simulink model "PeakDetect3"  (R2018b)
settings: Solver=FixedStepAuto  StartTime=0  StopTime=500*(15e-9)  FixedStep=15e-9  RelTol=1e-3
libraries: simulink x35, hdlsllib x34
(part 4 of 4)

== system PeakDetect3/xcorr_q1/Subsystem/Enabled Subsystem124 ==
  In1 : Inport
  Enable : EnablePort
  Out1 : Outport  InitialOutput=0
  wires:
  In1/1 -> Out1/1

== system PeakDetect3/xcorr_q1/Subsystem/Enabled Subsystem125 ==
  In1 : Inport
  Enable : EnablePort
  Out1 : Outport  InitialOutput=0
  wires:
  In1/1 -> Out1/1

== system PeakDetect3/xcorr_q1/Subsystem/Enabled Subsystem126 ==
  In1 : Inport
  Enable : EnablePort
  Out1 : Outport  InitialOutput=0
  wires:
  In1/1 -> Out1/1

== system PeakDetect3/xcorr_q1/Subsystem/Enabled Subsystem127 ==
  In1 : Inport
  Enable : EnablePort
  Out1 : Outport  InitialOutput=0
  wires:
  In1/1 -> Out1/1

== system PeakDetect3/xcorr_q1/Subsystem/Enabled Subsystem128 ==
  In1 : Inport
  Enable : EnablePort
  Out1 : Outport  InitialOutput=0
  wires:
  In1/1 -> Out1/1

== system PeakDetect3/xcorr_q1/Subsystem/Enabled Subsystem129 ==
  In1 : Inport
  Enable : EnablePort
  Out1 : Outport  InitialOutput=0
  wires:
  In1/1 -> Out1/1

== system PeakDetect3/xcorr_q1/Subsystem/Enabled Subsystem130 ==
  In1 : Inport
  Enable : EnablePort
  Out1 : Outport  InitialOutput=0
  wires:
  In1/1 -> Out1/1

== system PeakDetect3/xcorr_q1/Subsystem/Enabled Subsystem131 ==
  In1 : Inport
  Enable : EnablePort
  Out1 : Outport  InitialOutput=0
  wires:
  In1/1 -> Out1/1

== system PeakDetect3/xcorr_q1/Subsystem/Enabled Subsystem132 ==
  In1 : Inport
  Enable : EnablePort
  Out1 : Outport  InitialOutput=0
  wires:
  In1/1 -> Out1/1

== system PeakDetect3/xcorr_q1/Subsystem/Enabled Subsystem133 ==
  In1 : Inport
  Enable : EnablePort
  Out1 : Outport  InitialOutput=0
  wires:
  In1/1 -> Out1/1

== system PeakDetect3/xcorr_q1/Subsystem/Enabled Subsystem134 ==
  In1 : Inport
  Enable : EnablePort
  Out1 : Outport  InitialOutput=0
  wires:
  In1/1 -> Out1/1

== system PeakDetect3/xcorr_q1/Subsystem/Enabled Subsystem135 ==
  In1 : Inport
  Enable : EnablePort
  Out1 : Outport  InitialOutput=0
  wires:
  In1/1 -> Out1/1

== system PeakDetect3/xcorr_q1/Subsystem/Enabled Subsystem136 ==
  In1 : Inport
  Enable : EnablePort
  Out1 : Outport  InitialOutput=0
  wires:
  In1/1 -> Out1/1

== system PeakDetect3/xcorr_q1/Subsystem/Enabled Subsystem137 ==
  In1 : Inport
  Enable : EnablePort
  Out1 : Outport  InitialOutput=0
  wires:
  In1/1 -> Out1/1

== system PeakDetect3/xcorr_q1/Subsystem/Enabled Subsystem138 ==
  In1 : Inport
  Enable : EnablePort
  Out1 : Outport  InitialOutput=0
  wires:
  In1/1 -> Out1/1

== system PeakDetect3/xcorr_q1/Subsystem/Enabled Subsystem139 ==
  In1 : Inport
  Enable : EnablePort
  Out1 : Outport  InitialOutput=0
  wires:
  In1/1 -> Out1/1

== system PeakDetect3/xcorr_q1/Subsystem/Enabled Subsystem140 ==
  In1 : Inport
  Enable : EnablePort
  Out1 : Outport  InitialOutput=0
  wires:
  In1/1 -> Out1/1

== system PeakDetect3/xcorr_q1/Subsystem/Enabled Subsystem141 ==
  In1 : Inport
  Enable : EnablePort
  Out1 : Outport  InitialOutput=0
  wires:
  In1/1 -> Out1/1

== system PeakDetect3/xcorr_q1/Subsystem/Enabled Subsystem142 ==
  In1 : Inport
  Enable : EnablePort
  Out1 : Outport  InitialOutput=0
  wires:
  In1/1 -> Out1/1

== system PeakDetect3/xcorr_q1/Subsystem/Enabled Subsystem143 ==
  In1 : Inport
  Enable : EnablePort
  Out1 : Outport  InitialOutput=0
  wires:
  In1/1 -> Out1/1

== system PeakDetect3/xcorr_q1/Subsystem/Enabled Subsystem144 ==
  In1 : Inport
  Enable : EnablePort
  Out1 : Outport  InitialOutput=0
  wires:
  In1/1 -> Out1/1

== system PeakDetect3/xcorr_q1/Subsystem/Enabled Subsystem145 ==
  In1 : Inport
  Enable : EnablePort
  Out1 : Outport  InitialOutput=0
  wires:
  In1/1 -> Out1/1

== system PeakDetect3/xcorr_q1/Subsystem/Enabled Subsystem146 ==
  In1 : Inport
  Enable : EnablePort
  Out1 : Outport  InitialOutput=0
  wires:
  In1/1 -> Out1/1

== system PeakDetect3/xcorr_q1/Subsystem/Enabled Subsystem147 ==
  In1 : Inport
  Enable : EnablePort
  Out1 : Outport  InitialOutput=0
  wires:
  In1/1 -> Out1/1

== system PeakDetect3/xcorr_q1/Subsystem/Enabled Subsystem148 ==
  In1 : Inport
  Enable : EnablePort
  Out1 : Outport  InitialOutput=0
  wires:
  In1/1 -> Out1/1

== system PeakDetect3/xcorr_q1/Subsystem/Enabled Subsystem149 ==
  In1 : Inport
  Enable : EnablePort
  Out1 : Outport  InitialOutput=0
  wires:
  In1/1 -> Out1/1

== system PeakDetect3/xcorr_q1/Subsystem/Enabled Subsystem150 ==
  In1 : Inport
  Enable : EnablePort
  Out1 : Outport  InitialOutput=0
  wires:
  In1/1 -> Out1/1

== system PeakDetect3/xcorr_q1/Subsystem/Enabled Subsystem151 ==
  In1 : Inport
  Enable : EnablePort
  Out1 : Outport  InitialOutput=0
  wires:
  In1/1 -> Out1/1

== system PeakDetect3/xcorr_q1/Subsystem/Enabled Subsystem152 ==
  In1 : Inport
  Enable : EnablePort
  Out1 : Outport  InitialOutput=0
  wires:
  In1/1 -> Out1/1

== system PeakDetect3/xcorr_q1/Subsystem/Enabled Subsystem153 ==
  In1 : Inport
  Enable : EnablePort
  Out1 : Outport  InitialOutput=0
  wires:
  In1/1 -> Out1/1

== system PeakDetect3/xcorr_q1/Subsystem/Enabled Subsystem154 ==
  In1 : Inport
  Enable : EnablePort
  Out1 : Outport  InitialOutput=0
  wires:
  In1/1 -> Out1/1

== system PeakDetect3/xcorr_q1/Subsystem/Enabled Subsystem155 ==
  In1 : Inport
  Enable : EnablePort
  Out1 : Outport  InitialOutput=0
  wires:
  In1/1 -> Out1/1

== system PeakDetect3/xcorr_q1/Subsystem/Enabled Subsystem156 ==
  In1 : Inport
  Enable : EnablePort
  Out1 : Outport  InitialOutput=0
  wires:
  In1/1 -> Out1/1

== system PeakDetect3/xcorr_q1/Subsystem/Enabled Subsystem157 ==
  In1 : Inport
  Enable : EnablePort
  Out1 : Outport  InitialOutput=0
  wires:
  In1/1 -> Out1/1

== system PeakDetect3/xcorr_q1/Subsystem/Enabled Subsystem158 ==
  In1 : Inport
  Enable : EnablePort
  Out1 : Outport  InitialOutput=0
  wires:
  In1/1 -> Out1/1

== system PeakDetect3/xcorr_q1/Subsystem/Enabled Subsystem159 ==
  In1 : Inport
  Enable : EnablePort
  Out1 : Outport  InitialOutput=0
  wires:
  In1/1 -> Out1/1

== system PeakDetect3/xcorr_q1/Subsystem/Enabled Subsystem160 ==
  In1 : Inport
  Enable : EnablePort
  Out1 : Outport  InitialOutput=0
  wires:
  In1/1 -> Out1/1

== system PeakDetect3/xcorr_q1/Subsystem/Enabled Subsystem161 ==
  In1 : Inport
  Enable : EnablePort
  Out1 : Outport  InitialOutput=0
  wires:
  In1/1 -> Out1/1

== system PeakDetect3/xcorr_q1/Subsystem/Enabled Subsystem162 ==
  In1 : Inport
  Enable : EnablePort
  Out1 : Outport  InitialOutput=0
  wires:
  In1/1 -> Out1/1

== system PeakDetect3/xcorr_q1/Subsystem/Enabled Subsystem163 ==
  In1 : Inport
  Enable : EnablePort
  Out1 : Outport  InitialOutput=0
  wires:
  In1/1 -> Out1/1

== system PeakDetect3/xcorr_q1/Subsystem/Enabled Subsystem164 ==
  In1 : Inport
  Enable : EnablePort
  Out1 : Outport  InitialOutput=0
  wires:
  In1/1 -> Out1/1

== system PeakDetect3/xcorr_q1/Subsystem/Enabled Subsystem165 ==
  In1 : Inport
  Enable : EnablePort
  Out1 : Outport  InitialOutput=0
  wires:
  In1/1 -> Out1/1

== system PeakDetect3/xcorr_q1/Subsystem/Enabled Subsystem166 ==
  In1 : Inport
  Enable : EnablePort
  Out1 : Outport  InitialOutput=0
  wires:
  In1/1 -> Out1/1

== system PeakDetect3/xcorr_q1/Subsystem/Enabled Subsystem167 ==
  In1 : Inport
  Enable : EnablePort
  Out1 : Outport  InitialOutput=0
  wires:
  In1/1 -> Out1/1

== system PeakDetect3/xcorr_q1/Subsystem/Enabled Subsystem168 ==
  In1 : Inport
  Enable : EnablePort
  Out1 : Outport  InitialOutput=0
  wires:
  In1/1 -> Out1/1

== system PeakDetect3/xcorr_q1/Subsystem/Enabled Subsystem169 ==
  In1 : Inport
  Enable : EnablePort
  Out1 : Outport  InitialOutput=0
  wires:
  In1/1 -> Out1/1

== system PeakDetect3/xcorr_q1/Subsystem/Enabled Subsystem170 ==
  In1 : Inport
  Enable : EnablePort
  Out1 : Outport  InitialOutput=0
  wires:
  In1/1 -> Out1/1

== system PeakDetect3/xcorr_q1/Subsystem/Enabled Subsystem171 ==
  In1 : Inport
  Enable : EnablePort
  Out1 : Outport  InitialOutput=0
  wires:
  In1/1 -> Out1/1

== system PeakDetect3/xcorr_q1/Subsystem/Enabled Subsystem172 ==
  In1 : Inport
  Enable : EnablePort
  Out1 : Outport  InitialOutput=0
  wires:
  In1/1 -> Out1/1

== system PeakDetect3/xcorr_q1/Subsystem/Enabled Subsystem173 ==
  In1 : Inport
  Enable : EnablePort
  Out1 : Outport  InitialOutput=0
  wires:
  In1/1 -> Out1/1

== system PeakDetect3/xcorr_q1/Subsystem/Enabled Subsystem174 ==
  In1 : Inport
  Enable : EnablePort
  Out1 : Outport  InitialOutput=0
  wires:
  In1/1 -> Out1/1

== system PeakDetect3/xcorr_q1/Subsystem/Enabled Subsystem175 ==
  In1 : Inport
  Enable : EnablePort
  Out1 : Outport  InitialOutput=0
  wires:
  In1/1 -> Out1/1

== system PeakDetect3/xcorr_q1/Subsystem/Enabled Subsystem176 ==
  In1 : Inport
  Enable : EnablePort
  Out1 : Outport  InitialOutput=0
  wires:
  In1/1 -> Out1/1

== system PeakDetect3/xcorr_q1/Subsystem/Enabled Subsystem177 ==
  In1 : Inport
  Enable : EnablePort
  Out1 : Outport  InitialOutput=0
  wires:
  In1/1 -> Out1/1

== system PeakDetect3/xcorr_q1/Subsystem/Enabled Subsystem178 ==
  In1 : Inport
  Enable : EnablePort
  Out1 : Outport  InitialOutput=0
  wires:
  In1/1 -> Out1/1

== system PeakDetect3/xcorr_q1/Subsystem/Enabled Subsystem179 ==
  In1 : Inport
  Enable : EnablePort
  Out1 : Outport  InitialOutput=0
  wires:
  In1/1 -> Out1/1

== system PeakDetect3/xcorr_q1/Subsystem/Enabled Subsystem180 ==
  In1 : Inport
  Enable : EnablePort
  Out1 : Outport  InitialOutput=0
  wires:
  In1/1 -> Out1/1

== system PeakDetect3/xcorr_q1/Subsystem/Enabled Subsystem181 ==
  In1 : Inport
  Enable : EnablePort
  Out1 : Outport  InitialOutput=0
  wires:
  In1/1 -> Out1/1

== system PeakDetect3/xcorr_q1/Subsystem/Enabled Subsystem182 ==
  In1 : Inport
  Enable : EnablePort
  Out1 : Outport  InitialOutput=0
  wires:
  In1/1 -> Out1/1

== system PeakDetect3/xcorr_q1/Subsystem/Enabled Subsystem183 ==
  In1 : Inport
  Enable : EnablePort
  Out1 : Outport  InitialOutput=0
  wires:
  In1/1 -> Out1/1

== system PeakDetect3/xcorr_q1/Subsystem/Enabled Subsystem184 ==
  In1 : Inport
  Enable : EnablePort
  Out1 : Outport  InitialOutput=0
  wires:
  In1/1 -> Out1/1

== system PeakDetect3/xcorr_q1/Subsystem/Enabled Subsystem185 ==
  In1 : Inport
  Enable : EnablePort
  Out1 : Outport  InitialOutput=0
  wires:
  In1/1 -> Out1/1

== system PeakDetect3/xcorr_q1/Subsystem/Enabled Subsystem186 ==
  In1 : Inport
  Enable : EnablePort
  Out1 : Outport  InitialOutput=0
  wires:
  In1/1 -> Out1/1

== system PeakDetect3/xcorr_q1/Subsystem/Enabled Subsystem187 ==
  In1 : Inport
  Enable : EnablePort
  Out1 : Outport  InitialOutput=0
  wires:
  In1/1 -> Out1/1

== system PeakDetect3/xcorr_q1/Subsystem/Enabled Subsystem188 ==
  In1 : Inport
  Enable : EnablePort
  Out1 : Outport  InitialOutput=0
  wires:
  In1/1 -> Out1/1

== system PeakDetect3/xcorr_q1/Subsystem/Enabled Subsystem189 ==
  In1 : Inport
  Enable : EnablePort
  Out1 : Outport  InitialOutput=0
  wires:
  In1/1 -> Out1/1

== system PeakDetect3/xcorr_q1/Subsystem/Enabled Subsystem190 ==
  In1 : Inport
  Enable : EnablePort
  Out1 : Outport  InitialOutput=0
  wires:
  In1/1 -> Out1/1

== system PeakDetect3/xcorr_q1/Subsystem/Enabled Subsystem191 ==
  In1 : Inport
  Enable : EnablePort
  Out1 : Outport  InitialOutput=0
  wires:
  In1/1 -> Out1/1

== system PeakDetect3/xcorr_q1/Subsystem/Enabled Subsystem192 ==
  In1 : Inport
  Enable : EnablePort
  Out1 : Outport  InitialOutput=0
  wires:
  In1/1 -> Out1/1

== system PeakDetect3/xcorr_q1/Subsystem/Enabled Subsystem193 ==
  In1 : Inport
  Enable : EnablePort
  Out1 : Outport  InitialOutput=0
  wires:
  In1/1 -> Out1/1

== system PeakDetect3/xcorr_q1/Subsystem/Enabled Subsystem194 ==
  In1 : Inport
  Enable : EnablePort
  Out1 : Outport  InitialOutput=0
  wires:
  In1/1 -> Out1/1

== system PeakDetect3/xcorr_q1/Subsystem/Enabled Subsystem195 ==
  In1 : Inport
  Enable : EnablePort
  Out1 : Outport  InitialOutput=0
  wires:
  In1/1 -> Out1/1

== system PeakDetect3/xcorr_q1/Subsystem/Enabled Subsystem196 ==
  In1 : Inport
  Enable : EnablePort
  Out1 : Outport  InitialOutput=0
  wires:
  In1/1 -> Out1/1

== system PeakDetect3/xcorr_q1/Subsystem/Enabled Subsystem197 ==
  In1 : Inport
  Enable : EnablePort
  Out1 : Outport  InitialOutput=0
  wires:
  In1/1 -> Out1/1

== system PeakDetect3/xcorr_q1/Subsystem/Enabled Subsystem198 ==
  In1 : Inport
  Enable : EnablePort
  Out1 : Outport  InitialOutput=0
  wires:
  In1/1 -> Out1/1

== system PeakDetect3/xcorr_q1/Subsystem/Enabled Subsystem199 ==
  In1 : Inport
  Enable : EnablePort
  Out1 : Outport  InitialOutput=0
  wires:
  In1/1 -> Out1/1

== system PeakDetect3/xcorr_q1/Subsystem/Enabled Subsystem200 ==
  In1 : Inport
  Enable : EnablePort
  Out1 : Outport  InitialOutput=0
  wires:
  In1/1 -> Out1/1
